simulink model "sampleModel7214_pp_1_1_mu"  (R2018a)
settings: Solver=VariableStepAuto  StartTime=0.0  StopTime=10.0  RelTol=1e-3
undefined symbols (not defined in the file): DiscIntNeverNeededParam
libraries: simulink x52
(part 1 of 2)
settings Model: Creator=cyfuzz  LastModifiedBy=shafiul
settings CodeAppCC: StateflowObjectComments=on

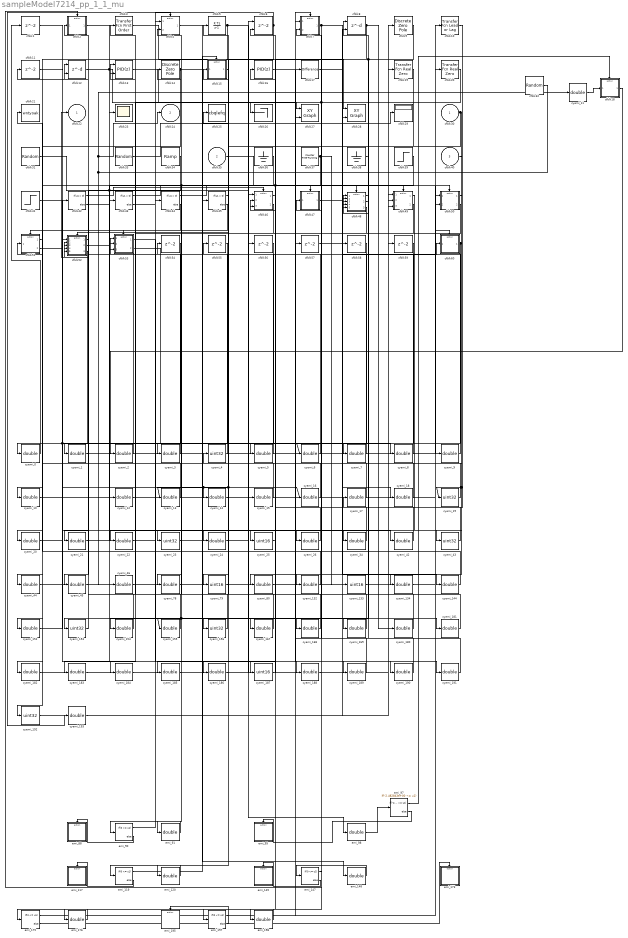
== system sampleModel7214_pp_1_1_mu ==
  cfblk30 : Inport
  cfblk35 : Inport  Port=2
  cfblk40 : Inport  Port=3
  cfblk{1,11,54..59} (8 alike) : Delay  SampleTime=1
  cfblk10 : simulink/Discrete/Transfer Fcn Lead or Lag  PoleZ=0.95  ZeroZ=0.75  ICPrevOutput=0.0  ICPrevInput=0.0  DoSatur=off
      settings: SourceProductName=Simulink  SourceProductBaseCode=SL
  cfblk12 : Delay  DelayLengthSource=Input port  SampleTime=1
      settings: InputPortMap=u0,p1
  cfblk13 : simulink/Continuous/PID Controller (2DOF)  Controller=PID  TimeDomain=Discrete-time  SampleTime=1  IntegratorMethod=Forward Euler  FilterMethod=Forward Euler  Form=Parallel  UseFilter=on  ControllerParametersSource=internal  P=1  I=1  D=0  N=100  b=1  c=1  InitialConditionSource=internal  InitialConditionForIntegrator=0  InitialConditionForFilter=0  ExternalReset=none  LimitOutput=off  UpperSaturationLimit=inf  LowerSaturationLimit=-inf  LinearizeAsGain=off  AntiWindupMode=none  Kb=1  TrackingMode=off  Kt=1  PParamMin=[]  PParamMax=[]  IParamMin=[]  IParamMax=[]  DParamMin=[]  DParamMax=[]  NParamMin=[]  NParamMax=[]  bParamMin=[]  bParamMax=[]  cParamMin=[]  cParamMax=[]  KbParamMin=[]  KbParamMax=[]  KtParamMin=[]  KtParamMax=[]  POutMin=[]  POutMax=[]  IOutMin=[]  IOutMax=[]  DOutMin=[]  DOutMax=[]  NOutMin=[]  NOutMax=[]  bOutMin=[]  bOutMax=[]  cOutMin=[]  cOutMax=[]  KbOutMin=[]  KbOutMax=[]  KtOutMin=[]  KtOutMax=[]  IntegratorOutMin=[]  IntegratorOutMax=[]  FilterOutMin=[]  FilterOutMax=[]  SumOutMin=[]  SumOutMax=[]  Sum1OutMin=[]  Sum1OutMax=[]  Sum2OutMin=[]  Sum2OutMax=[]  Sum3OutMin=[]  Sum3OutMax=[]  SumI1OutMin=[]  SumI1OutMax=[]  SumI2OutMin=[]  SumI2OutMax=[]  SumI3OutMin=[]  SumI3OutMax=[]  SumDOutMin=[]  SumDOutMax=[]  SaturationOutMin=[]  SaturationOutMax=[]  IntegratorContinuousStateAttributes=''  IntegratorStateMustResolveToSignalObject=off  IntegratorRTWStateStorageClass=Auto  FilterContinuousStateAttributes=''  FilterStateMustResolveToSignalObject=off  FilterRTWStateStorageClass=Auto  DifferentiatorICPrevScaledInput=0  DifferentiatorOutMin=[]  DifferentiatorOutMax=[]  FilterDiffOutCoefMin=[]  FilterDiffOutCoefMax=[]  SumDenOutMin=[]  SumDenOutMax=[]  SumNumOutMin=[]  SumNumOutMax=[]  ReciprocalOutMin=[]  ReciprocalOutMax=[]  DivideOutMin=[]  DivideOutMax=[]  TunerSelectOption=Transfer Function Based (PID Tuner App)
  cfblk14 : DiscreteZeroPole  Poles=[0 0.5]  Gain=1
  cfblk15 : Subsystem  TreatAsAtomicUnit=on
  cfblk16 : simulink/Continuous/PID Controller  Controller=PID  TimeDomain=Discrete-time  SampleTime=1  IntegratorMethod=Forward Euler  FilterMethod=Forward Euler  Form=Parallel  UseFilter=on  ControllerParametersSource=internal  P=1  I=1  D=0  N=100  InitialConditionSource=internal  InitialConditionForIntegrator=0  InitialConditionForFilter=0  ExternalReset=none  LimitOutput=off  UpperSaturationLimit=inf  LowerSaturationLimit=-inf  LinearizeAsGain=off  AntiWindupMode=none  Kb=1  TrackingMode=off  Kt=1  PParamMin=[]  PParamMax=[]  IParamMin=[]  IParamMax=[]  DParamMin=[]  DParamMax=[]  NParamMin=[]  NParamMax=[]  KbParamMin=[]  KbParamMax=[]  KtParamMin=[]  KtParamMax=[]  POutMin=[]  POutMax=[]  IOutMin=[]  IOutMax=[]  DOutMin=[]  DOutMax=[]  NOutMin=[]  NOutMax=[]  KbOutMin=[]  KbOutMax=[]  KtOutMin=[]  KtOutMax=[]  IntegratorOutMin=[]  IntegratorOutMax=[]  FilterOutMin=[]  FilterOutMax=[]  SumOutMin=[]  SumOutMax=[]  SumI1OutMin=[]  SumI1OutMax=[]  SumI2OutMin=[]  SumI2OutMax=[]  SumI3OutMin=[]  SumI3OutMax=[]  SumDOutMin=[]  SumDOutMax=[]  SaturationOutMin=[]  SaturationOutMax=[]  IntegratorContinuousStateAttributes=''  IntegratorStateMustResolveToSignalObject=off  IntegratorRTWStateStorageClass=Auto  FilterContinuousStateAttributes=''  FilterStateMustResolveToSignalObject=off  FilterRTWStateStorageClass=Auto  DifferentiatorICPrevScaledInput=0  DifferentiatorOutMin=[]  DifferentiatorOutMax=[]  FilterDiffOutCoefMin=[]  FilterDiffOutCoefMax=[]  SumDenOutMin=[]  SumDenOutMax=[]  SumNumOutMin=[]  SumNumOutMax=[]  ReciprocalOutMin=[]  ReciprocalOutMax=[]  DivideOutMin=[]  DivideOutMax=[]  TunerSelectOption=Transfer Function Based (PID Tuner App)
  cfblk17 : simulink/Discrete/Difference  ICPrevInput=0.0  OutMin=[]  OutMax=[]  OutDataTypeStr=double  OutputDataTypeScalingMode=double  OutDataType=fixdt(1, 16)  OutScaling=2^-10  DoSatur=off
  cfblk18 : Subsystem  TreatAsAtomicUnit=on
  cfblk19 : simulink/Discrete/Transfer Fcn Real Zero  ZeroZ=0.75  ICPrevInput=0.0  DoSatur=off
      settings: SourceProductName=Simulink  SourceProductBaseCode=SL
  cfblk2 : Subsystem  TreatAsAtomicUnit=on
  cfblk20 : simulink/Discrete/Transfer Fcn Real Zero  ZeroZ=0.75  ICPrevInput=0.0  DoSatur=off
      settings: SourceProductName=Simulink  SourceProductBaseCode=SL
  cfblk21 : ToWorkspace  VariableName=wntyoak  SaveFormat=Timeseries  SampleTime=-1
  cfblk23 : Scope
  cfblk25 : ToWorkspace  VariableName=cbqlefq  SaveFormat=Timeseries  SampleTime=-1
  cfblk26 : Terminator
  cfblk27 : simulink/Sinks/XY Graph  xmin=-1  xmax=1  ymin=-1  ymax=1  st=-1
  cfblk28 : simulink/Sinks/XY Graph  xmin=-1  xmax=1  ymin=-1  ymax=1  st=-1
  cfblk29 : Display
  cfblk3 : simulink/Discrete/Transfer Fcn First Order  PoleZ=0.95  ICPrevOutput=0.0  DoSatur=off
      settings: SourceProductName=Simulink
  cfblk31 : RandomNumber  SampleTime=0.1
  cfblk32 : RandomNumber  SampleTime=0.1
  cfblk33 : UniformRandomNumber  SampleTime=0.1
  cfblk34 : simulink/Sources/Ramp  slope=1  start=0  InitialOutput=0
  cfblk36 : Ground
  cfblk37 : simulink/Sources/Counter Free-Running  NumBits=16  tsamp=1
  cfblk38 : Ground
  cfblk39 : Step  After=69  SampleTime=0
  cfblk4 : Subsystem  TreatAsAtomicUnit=on
  cfblk41 : Step  After=79  SampleTime=0
  cfblk{42..45} (4 alike) : If  SampleTime=1
  cfblk46 : Subsystem  TreatAsAtomicUnit=on
  cfblk47 : Subsystem  TreatAsAtomicUnit=on
  cfblk48 : Subsystem  TreatAsAtomicUnit=on
  cfblk49 : Subsystem  TreatAsAtomicUnit=on
  cfblk5 : DiscreteIntegrator  OutDataTypeStr=double  ICPrevOutput=DiscIntNeverNeededParam  ICPrevScaledInput=DiscIntNeverNeededParam
  cfblk50 : Subsystem  TreatAsAtomicUnit=on
  cfblk51 : Subsystem  TreatAsAtomicUnit=on
  cfblk52 : Subsystem  TreatAsAtomicUnit=on
  cfblk53 : Subsystem  TreatAsAtomicUnit=on
  cfblk6 : Delay  ShowEnablePort=on  SampleTime=1
      settings: InputPortMap=u0,e6
  cfblk60 : Subsystem  TreatAsAtomicUnit=on
  cfblk7 : Subsystem  TreatAsAtomicUnit=on
  cfblk8 : Delay  DelayLengthSource=Input port  SampleTime=1
      settings: InputPortMap=u0,p1
  cfblk9 : DiscreteZeroPole  Poles=[0 0.5]  Gain=1
  cyemi_{0..3,5..18,20..22,24,26,34,42,44..46,78,80,132,134,144,152,154..155,167..169,180..186,188..191,193} (51 alike) : DataTypeConversion  OutDataTypeStr=double
  cyemi_{25,79,133,187} (4 alike) : DataTypeConversion  OutDataTypeStr=uint16
  cyemi_{4,19,23,43,153,156,192} (7 alike) : DataTypeConversion  OutDataTypeStr=uint32
  emi_117 : Subsystem  TreatAsAtomicUnit=on
  emi_{90,119,147,175,197} (5 alike) : If  IfExpression=0 <= u1
  emi_{91,98,120,148,176,198} (6 alike) : DataTypeConversion  OutDataTypeStr=double
  emi_145 : Subsystem  TreatAsAtomicUnit=on
  emi_173 : Subsystem  TreatAsAtomicUnit=on
  emi_195 : Subsystem  TreatAsAtomicUnit=on
  emi_88 : Subsystem  TreatAsAtomicUnit=on
  emi_95 : Subsystem  TreatAsAtomicUnit=on
  emi_97 : If  IfExpression=-2.482843e+00 <= u1  SampleTime=1
  cfblk22 : Outport
  cfblk24 : Outport  Port=2
  wires:
  cfblk52/1(cfblk2) -> cfblk22/1
  cfblk37/1 -> cyemi_79/1, cyemi_187/1, cyemi_133/1
  cfblk3/1 -> cfblk28/1
  cfblk13/1 -> cfblk26/1
  cfblk20/1 -> cyemi_132/1, cyemi_154/1
  cfblk32/1 -> cyemi_11/1, cfblk24/1, cyemi_46/1
  cfblk9/1 -> cyemi_5/1, cyemi_7/1
  cfblk8/1 -> cfblk27/1, cyemi_180/1
  cfblk36/1 -> cyemi_23/1, cyemi_192/1
  cfblk41/1 -> cyemi_14/1, cyemi_16/1, cyemi_6/1
  cfblk5/1 -> cyemi_34/1, cyemi_44/1
  cfblk12/1 -> cfblk27/2, cyemi_188/1
  cfblk33/1 -> cfblk29/1
  cfblk30/1 -> cyemi_19/1, cyemi_43/1, cyemi_156/1
  cfblk42/1 -> cfblk46/Action
  cfblk42/2 -> cfblk47/Action
  cfblk43/1 -> cfblk48/Action
  cfblk43/2 -> cfblk49/Action
  cfblk44/1 -> cfblk50/Action
  cfblk44/2 -> cfblk51/Action
  cfblk45/1 -> cfblk52/Action
  cfblk45/2 -> cfblk53/Action
  cyemi_0/1 -> cfblk1/1
  cfblk58/1 -> cyemi_0/1
  cyemi_1/1 -> cfblk10/1
  cfblk34/1 -> cyemi_1/1
  cyemi_2/1 -> cfblk11/1
  cyemi_3/1 -> cfblk12/1
  cfblk51/2(cfblk8) -> cyemi_3/1
  cyemi_4/1 -> cfblk12/2
  cfblk40/1 -> cyemi_4/1
  cyemi_5/1 -> cfblk13/1
  cyemi_6/1 -> cfblk13/2
  cyemi_7/1 -> cfblk14/1
  cyemi_9/1 -> cfblk16/1
  cfblk35/1 -> cyemi_9/1
  cyemi_10/1 -> cfblk17/1
  cfblk51/1(cfblk2) -> cyemi_10/1
  cyemi_12/1 -> cfblk19/1
  cfblk31/1 -> cyemi_12/1, emi_98/1
  cyemi_14/1 -> cfblk20/1
  cyemi_15/1 -> cfblk21/1
  cfblk53/2(cfblk11) -> cyemi_15/1
  cyemi_16/1 -> cfblk25/1
  cyemi_17/1 -> cfblk3/1
  cfblk10/1 -> cyemi_17/1
  cfblk17/1 -> cyemi_18/1
  cyemi_20/1 -> cfblk42/1
  cfblk52/3(cfblk15) -> cyemi_20/1
  cyemi_21/1 -> cfblk43/1
  cfblk55/1 -> cyemi_21/1
  cyemi_22/1 -> cfblk44/1
  cfblk49/1(cfblk2) -> cyemi_22/1
  cyemi_23/1 -> cfblk45/1
  cyemi_24/1 -> cfblk46/1(cfblk1)
  cfblk49/2(cfblk16) -> cyemi_24/1
  cyemi_25/1 -> cfblk46/2(cfblk9)
  cfblk50/1(cfblk2) -> cyemi_25/1
  cyemi_26/1 -> cfblk46/3(cfblk10)
  cfblk19/1 -> cyemi_26/1
  cyemi_34/1 -> cfblk47/1(cfblk1)
  cyemi_42/1 -> cfblk48/1(cfblk1)
  cfblk1/1 -> cyemi_42/1
  cyemi_43/1 -> cfblk48/2(cfblk10)
  cyemi_44/1 -> cfblk48/3(cfblk11)
  cyemi_45/1 -> cfblk48/4(cfblk12)
  cfblk54/1 -> cyemi_45/1
  cyemi_46/1 -> cfblk48/5(cfblk13)
  cyemi_78/1 -> cfblk49/1(cfblk1)
  cfblk48/3(cfblk15) -> cyemi_78/1
  cyemi_79/1 -> cfblk49/2(cfblk14)
  cyemi_80/1 -> cfblk49/3(cfblk15)
  cyemi_132/1 -> cfblk5/1
  cyemi_133/1 -> cfblk50/1(cfblk1)
  cyemi_134/1 -> cfblk50/2(cfblk12)
  cfblk57/1 -> cyemi_134/1
  cyemi_144/1 -> cfblk51/1(cfblk1)
  cfblk47/1(cfblk2) -> cyemi_144/1
  cyemi_152/1 -> cfblk52/1(cfblk1)
  cfblk56/1 -> cyemi_152/1
  cyemi_153/1 -> cfblk52/2(cfblk10)
  cfblk48/2(cfblk14) -> cyemi_153/1
  cyemi_154/1 -> cfblk52/3(cfblk11)
  cyemi_155/1 -> cfblk52/4(cfblk12)
  cfblk59/1 -> cyemi_155/1, emi_91/1
  cyemi_156/1 -> cfblk52/5(cfblk13)
  cyemi_167/1 -> cfblk53/1(cfblk1)
  cfblk48/1(cfblk2) -> cyemi_167/1
  cyemi_168/1 -> cfblk53/2(cfblk9)
  cfblk39/1 -> cyemi_168/1
  cyemi_169/1 -> cfblk53/3(cfblk10)
  cfblk38/1 -> cyemi_169/1
  cyemi_180/1 -> cfblk54/1
  cyemi_181/1 -> cfblk55/1
  cfblk52/2(cfblk14) -> cyemi_181/1
  cyemi_182/1 -> cfblk56/1
  cfblk14/1 -> cyemi_182/1, emi_148/1
  cyemi_183/1 -> cfblk57/1
  cfblk46/2(cfblk11) -> cyemi_183/1
  cyemi_184/1 -> cfblk58/1
  cfblk50/2(cfblk13) -> cyemi_184/1
  cyemi_185/1 -> cfblk59/1
  cyemi_186/1 -> cfblk6/1
  cfblk46/1(cfblk2) -> cyemi_186/1
  cyemi_187/1 -> cfblk6/2
  cfblk11/1 -> cyemi_189/1
  cfblk16/1 -> cyemi_190/1
  cyemi_191/1 -> cfblk8/1
  cfblk53/1(cfblk2) -> cyemi_191/1
  cyemi_192/1 -> cfblk8/2
  cyemi_193/1 -> cfblk9/1
  cfblk6/1 -> cyemi_193/1, emi_120/1
  cyemi_18/1 -> cfblk4/1(emi_85)
  cyemi_19/1 -> cfblk4/2(emi_86)
  cfblk4/1(emi_87) -> cyemi_8/1
  emi_90/1 -> cfblk4/Action
  emi_90/2 -> emi_88/Action
  emi_91/1 -> emi_90/1
  cyemi_11/1 -> cfblk18/1(emi_93)
  cfblk18/1(emi_94) -> cyemi_2/1
  emi_97/1 -> cfblk18/Action
  emi_97/2 -> emi_95/Action
  emi_98/1 -> emi_97/1
  cyemi_8/1 -> cfblk15/1(emi_115)
  cfblk15/1(emi_116) -> cyemi_185/1, cyemi_13/1
  emi_119/1 -> cfblk15/Action
  emi_119/2 -> emi_117/Action
  emi_120/1 -> emi_119/1
  cyemi_13/1 -> cfblk2/1(emi_143)
  cfblk2/1(emi_144) -> cfblk23/1
  emi_147/1 -> cfblk2/Action
  emi_147/2 -> emi_145/Action
  emi_148/1 -> emi_147/1
  cyemi_188/1 -> cfblk60/1(emi_171)
  cfblk60/1(emi_172) -> cyemi_80/1, emi_198/1
  emi_175/1 -> cfblk60/Action
  emi_175/2 -> emi_173/Action
  emi_176/1 -> emi_175/1
  cyemi_189/1 -> cfblk7/1(emi_192)
  cyemi_190/1 -> cfblk7/2(emi_193)
  cfblk7/1(emi_194) -> emi_176/1, cfblk28/2
  emi_197/1 -> cfblk7/Action
  emi_197/2 -> emi_195/Action
  emi_198/1 -> emi_197/1

== system sampleModel7214_pp_1_1_mu/cfblk15 ==
  emi_115 : Inport
  Action Port : ActionPort  ActionType=then
  cfblk15 : simulink/Discrete/Transfer Fcn Real Zero  ZeroZ=0.75  ICPrevInput=0.0  DoSatur=off
      settings: SourceProductName=Simulink  SourceProductBaseCode=SL
  emi_116 : Outport
  wires:
  emi_115/1 -> cfblk15/1
  cfblk15/1 -> emi_116/1

== system sampleModel7214_pp_1_1_mu/cfblk18 ==
  emi_93 : Inport
  Action Port : ActionPort  ActionType=then
  cfblk18 : UnitDelay
  emi_94 : Outport
  wires:
  emi_93/1 -> cfblk18/1
  cfblk18/1 -> emi_94/1

== system sampleModel7214_pp_1_1_mu/cfblk2 ==
  emi_143 : Inport
  Action Port : ActionPort  ActionType=then
  cfblk2 : simulink/Discrete/Difference  ICPrevInput=0.0  OutMin=[]  OutMax=[]  OutDataTypeStr=double  OutputDataTypeScalingMode=double  OutDataType=fixdt(1, 16)  OutScaling=2^-10  DoSatur=off
  emi_144 : Outport
  wires:
  emi_143/1 -> cfblk2/1
  cfblk2/1 -> emi_144/1

== system sampleModel7214_pp_1_1_mu/cfblk4 ==
  emi_85 : Inport
  emi_86 : Inport  Port=2
  Action Port : ActionPort  ActionType=then
  cfblk4 : Delay  ShowEnablePort=on  SampleTime=1
      settings: InputPortMap=u0,e6
  emi_87 : Outport
  wires:
  emi_85/1 -> cfblk4/1
  emi_86/1 -> cfblk4/2
  cfblk4/1 -> emi_87/1

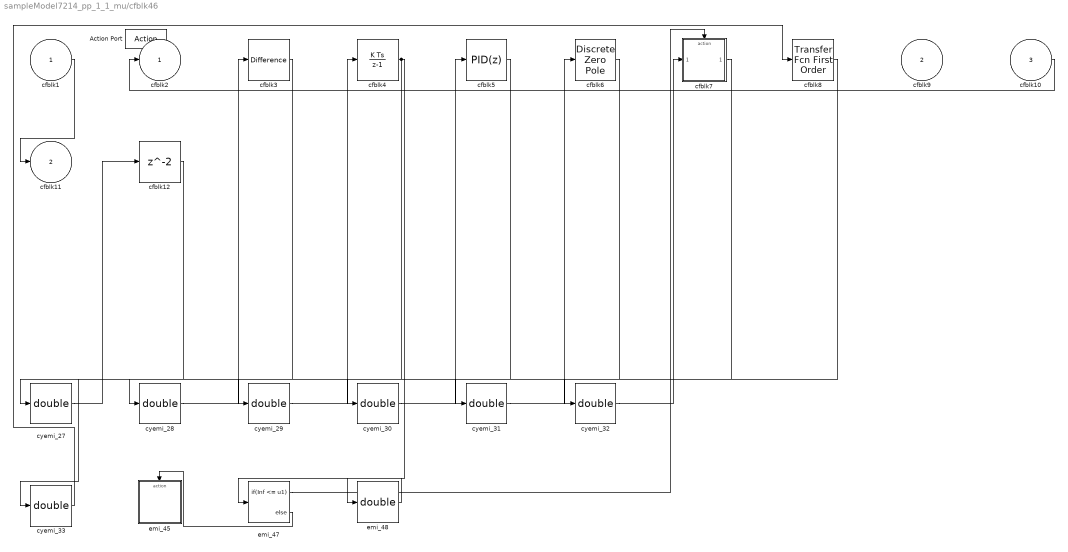
== system sampleModel7214_pp_1_1_mu/cfblk46 ==
  cfblk1 : Inport
  cfblk9 : Inport  Port=2
  cfblk10 : Inport  Port=3
  Action Port : ActionPort  ActionType=then
  cfblk12 : Delay
  cfblk3 : simulink/Discrete/Difference  ICPrevInput=0.0  OutMin=[]  OutMax=[]  OutDataTypeStr=double  OutputDataTypeScalingMode=double  OutDataType=fixdt(1, 16)  OutScaling=2^-10  DoSatur=off
  cfblk4 : DiscreteIntegrator  SampleTime=-1  OutDataTypeStr=double  ICPrevOutput=DiscIntNeverNeededParam  ICPrevScaledInput=DiscIntNeverNeededParam
  cfblk5 : simulink/Continuous/PID Controller  Controller=PID  TimeDomain=Discrete-time  SampleTime=-1  IntegratorMethod=Forward Euler  FilterMethod=Forward Euler  Form=Parallel  UseFilter=on  ControllerParametersSource=internal  P=1  I=1  D=0  N=100  InitialConditionSource=internal  InitialConditionForIntegrator=0  InitialConditionForFilter=0  ExternalReset=none  LimitOutput=off  UpperSaturationLimit=inf  LowerSaturationLimit=-inf  LinearizeAsGain=off  AntiWindupMode=none  Kb=1  TrackingMode=off  Kt=1  PParamMin=[]  PParamMax=[]  IParamMin=[]  IParamMax=[]  DParamMin=[]  DParamMax=[]  NParamMin=[]  NParamMax=[]  KbParamMin=[]  KbParamMax=[]  KtParamMin=[]  KtParamMax=[]  POutMin=[]  POutMax=[]  IOutMin=[]  IOutMax=[]  DOutMin=[]  DOutMax=[]  NOutMin=[]  NOutMax=[]  KbOutMin=[]  KbOutMax=[]  KtOutMin=[]  KtOutMax=[]  IntegratorOutMin=[]  IntegratorOutMax=[]  FilterOutMin=[]  FilterOutMax=[]  SumOutMin=[]  SumOutMax=[]  SumI1OutMin=[]  SumI1OutMax=[]  SumI2OutMin=[]  SumI2OutMax=[]  SumI3OutMin=[]  SumI3OutMax=[]  SumDOutMin=[]  SumDOutMax=[]  SaturationOutMin=[]  SaturationOutMax=[]  IntegratorContinuousStateAttributes=''  IntegratorStateMustResolveToSignalObject=off  IntegratorRTWStateStorageClass=Auto  FilterContinuousStateAttributes=''  FilterStateMustResolveToSignalObject=off  FilterRTWStateStorageClass=Auto  DifferentiatorICPrevScaledInput=0  DifferentiatorOutMin=[]  DifferentiatorOutMax=[]  FilterDiffOutCoefMin=[]  FilterDiffOutCoefMax=[]  SumDenOutMin=[]  SumDenOutMax=[]  SumNumOutMin=[]  SumNumOutMax=[]  ReciprocalOutMin=[]  ReciprocalOutMax=[]  DivideOutMin=[]  DivideOutMax=[]  TunerSelectOption=Transfer Function Based (PID Tuner App)
  cfblk6 : DiscreteZeroPole  Poles=[0 0.5]  Gain=1  SampleTime=-1
  cfblk7 : Subsystem  TreatAsAtomicUnit=on
  cfblk8 : simulink/Discrete/Transfer Fcn First Order  PoleZ=0.95  ICPrevOutput=0.0  DoSatur=off
      settings: SourceProductName=Simulink
  cyemi_{27..33} (7 alike) : DataTypeConversion  OutDataTypeStr=double
  emi_45 : Subsystem  TreatAsAtomicUnit=on
  emi_47 : If  IfExpression=Inf <= u1
  emi_48 : DataTypeConversion  OutDataTypeStr=double
  cfblk2 : Outport
  cfblk11 : Outport  Port=2
  wires:
  cfblk10/1 -> cfblk2/1
  cfblk1/1 -> cfblk11/1
  cyemi_27/1 -> cfblk12/1
  cfblk5/1 -> cyemi_27/1
  cyemi_28/1 -> cfblk3/1
  cfblk12/1 -> cyemi_28/1
  cyemi_29/1 -> cfblk4/1
  cyemi_30/1 -> cfblk5/1
  cfblk4/1 -> cyemi_30/1, emi_48/1
  cyemi_31/1 -> cfblk6/1
  cfblk8/1 -> cyemi_31/1
  cfblk6/1 -> cyemi_32/1
  cyemi_33/1 -> cfblk8/1
  cfblk3/1 -> cyemi_33/1
  cyemi_32/1 -> cfblk7/1(emi_43)
  cfblk7/1(emi_44) -> cyemi_29/1
  emi_47/1 -> cfblk7/Action
  emi_47/2 -> emi_45/Action
  emi_48/1 -> emi_47/1

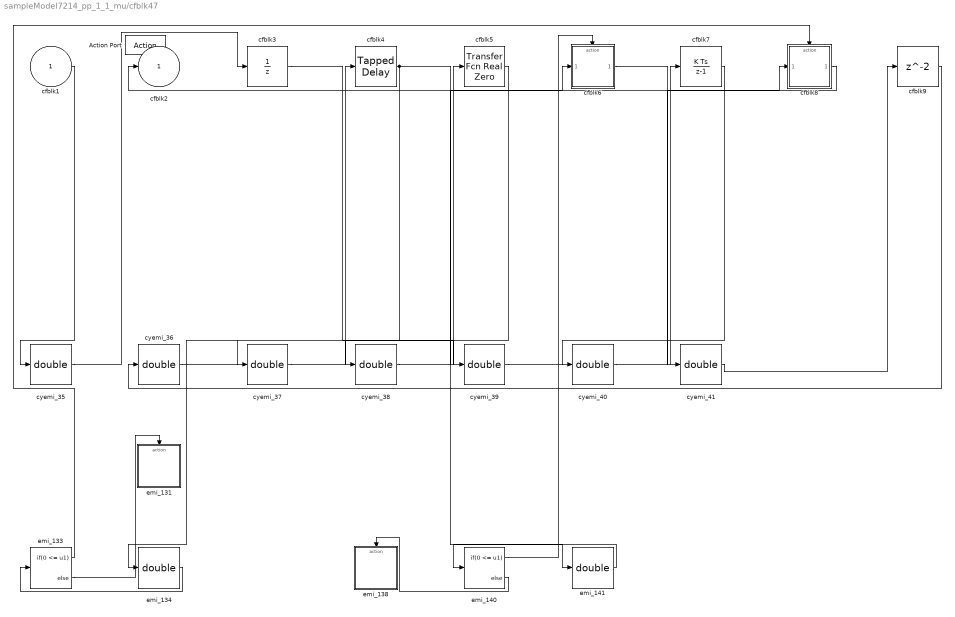
== system sampleModel7214_pp_1_1_mu/cfblk47 ==
  cfblk1 : Inport
  Action Port : ActionPort  ActionType=else
  cfblk3 : UnitDelay  SampleTime=-1
  cfblk4 : simulink/Discrete/Tapped Delay  vinit=0.0  samptime=-1  NumDelays=1  DelayOrder=Oldest  includeCurrent=off
  cfblk5 : simulink/Discrete/Transfer Fcn Real Zero  ZeroZ=0.75  ICPrevInput=0.0  DoSatur=off
      settings: SourceProductName=Simulink  SourceProductBaseCode=SL
  cfblk6 : Subsystem  TreatAsAtomicUnit=on
  cfblk7 : DiscreteIntegrator  SampleTime=-1  OutDataTypeStr=double  ICPrevOutput=DiscIntNeverNeededParam  ICPrevScaledInput=DiscIntNeverNeededParam
  cfblk8 : Subsystem  TreatAsAtomicUnit=on
  cfblk9 : Delay
  cyemi_{35..41} (7 alike) : DataTypeConversion  OutDataTypeStr=double
  emi_131 : Subsystem  TreatAsAtomicUnit=on
  emi_133 : If  IfExpression=0 <= u1
  emi_134 : DataTypeConversion  OutDataTypeStr=double
  emi_138 : Subsystem  TreatAsAtomicUnit=on
  emi_140 : If  IfExpression=0 <= u1
  emi_141 : DataTypeConversion  OutDataTypeStr=double
  cfblk2 : Outport
  wires:
  cyemi_35/1 -> cfblk3/1
  cfblk1/1 -> cyemi_35/1
  cyemi_36/1 -> cfblk4/1
  cfblk9/1 -> cyemi_36/1
  cyemi_37/1 -> cfblk5/1
  cfblk4/1 -> cyemi_37/1, emi_134/1, emi_141/1
  cfblk5/1 -> cyemi_38/1
  cyemi_39/1 -> cfblk7/1
  cfblk3/1 -> cyemi_39/1
  cfblk7/1 -> cyemi_40/1
  cyemi_41/1 -> cfblk9/1
  cyemi_40/1 -> cfblk8/1(emi_129)
  cfblk8/1(emi_130) -> cfblk2/1
  emi_133/1 -> cfblk8/Action
  emi_133/2 -> emi_131/Action
  emi_134/1 -> emi_133/1
  cyemi_38/1 -> cfblk6/1(emi_136)
  cfblk6/1(emi_137) -> cyemi_41/1
  emi_140/1 -> cfblk6/Action
  emi_140/2 -> emi_138/Action
  emi_141/1 -> emi_140/1

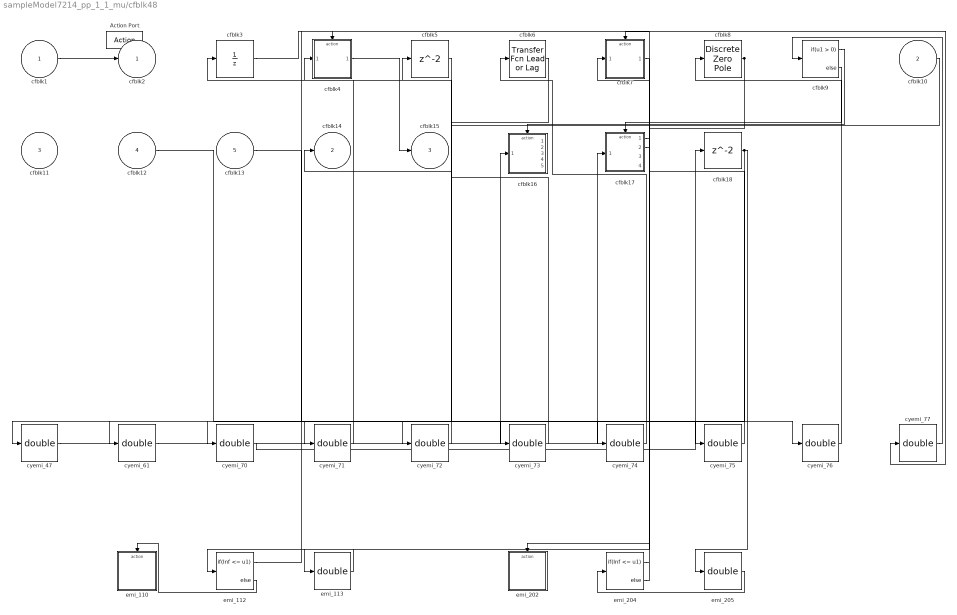
== system sampleModel7214_pp_1_1_mu/cfblk48 ==
  cfblk1 : Inport
  cfblk10 : Inport  Port=2
  cfblk11 : Inport  Port=3
  cfblk12 : Inport  Port=4
  cfblk13 : Inport  Port=5
  Action Port : ActionPort  ActionType=then
  cfblk16 : Subsystem  TreatAsAtomicUnit=on
  cfblk17 : Subsystem  TreatAsAtomicUnit=on
  cfblk18 : Delay
  cfblk3 : UnitDelay  SampleTime=-1
  cfblk4 : Subsystem  TreatAsAtomicUnit=on
  cfblk5 : Delay
  cfblk6 : simulink/Discrete/Transfer Fcn Lead or Lag  PoleZ=0.95  ZeroZ=0.75  ICPrevOutput=0.0  ICPrevInput=0.0  DoSatur=off
      settings: SourceProductName=Simulink  SourceProductBaseCode=SL
  cfblk7 : Subsystem  TreatAsAtomicUnit=on
  cfblk8 : DiscreteZeroPole  Poles=[0 0.5]  Gain=1  SampleTime=-1
  cfblk9 : If  SampleTime=1
  cyemi_{47,61,70..77} (10 alike) : DataTypeConversion  OutDataTypeStr=double
  emi_110 : Subsystem  TreatAsAtomicUnit=on
  emi_112 : If  IfExpression=Inf <= u1
  emi_113 : DataTypeConversion  OutDataTypeStr=double
  emi_202 : Subsystem  TreatAsAtomicUnit=on
  emi_204 : If  IfExpression=Inf <= u1
  emi_205 : DataTypeConversion  OutDataTypeStr=double
  cfblk2 : Outport
  cfblk14 : Outport  Port=2
  cfblk15 : Outport  Port=3
  wires:
  cfblk10/1 -> cfblk14/1
  cfblk1/1 -> cfblk2/1
  cfblk9/1 -> cfblk16/Action
  cfblk9/2 -> cfblk17/Action
  cyemi_47/1 -> cfblk16/1(cfblk1)
  cfblk17/1(cfblk2) -> cyemi_47/1
  cyemi_61/1 -> cfblk17/1(cfblk1)
  cfblk8/1 -> cyemi_61/1, emi_113/1
  cyemi_70/1 -> cfblk18/1
  cfblk5/1 -> cyemi_70/1
  cyemi_71/1 -> cfblk3/1
  cfblk18/1 -> cyemi_71/1, emi_205/1
  cfblk6/1 -> cyemi_72/1
  cyemi_73/1 -> cfblk5/1
  cfblk17/2(cfblk9) -> cyemi_73/1
  cyemi_74/1 -> cfblk6/1
  cfblk12/1 -> cyemi_75/1
  cyemi_76/1 -> cfblk8/1
  cfblk13/1 -> cyemi_76/1
  cyemi_77/1 -> cfblk9/1
  cfblk3/1 -> cyemi_77/1
  cyemi_72/1 -> cfblk4/1(emi_108)
  cfblk4/1(emi_109) -> cfblk15/1
  emi_112/1 -> cfblk4/Action
  emi_112/2 -> emi_110/Action
  emi_113/1 -> emi_112/1
  cyemi_75/1 -> cfblk7/1(emi_200)
  cfblk7/1(emi_201) -> cyemi_74/1
  emi_204/1 -> cfblk7/Action
  emi_204/2 -> emi_202/Action
  emi_205/1 -> emi_204/1

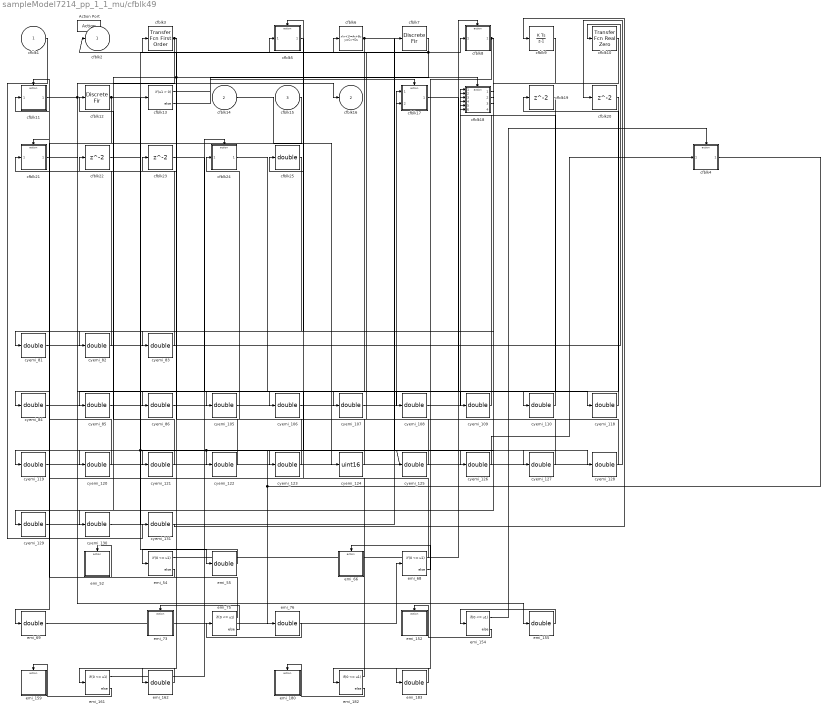
== system sampleModel7214_pp_1_1_mu/cfblk49 ==
  cfblk1 : Inport
  cfblk14 : Inport  Port=2
  cfblk15 : Inport  Port=3
  Action Port : ActionPort  ActionType=else
  cfblk10 : simulink/Discrete/Transfer Fcn Real Zero  ZeroZ=0.75  ICPrevInput=0.0  DoSatur=off
      settings: SourceProductName=Simulink  SourceProductBaseCode=SL
  cfblk11 : Subsystem  TreatAsAtomicUnit=on
  cfblk12 : DiscreteFir
  cfblk13 : If  SampleTime=1
  cfblk17 : Subsystem  TreatAsAtomicUnit=on
  cfblk18 : Subsystem  TreatAsAtomicUnit=on
  cfblk{19..20,22..23} (4 alike) : Delay
  cfblk21 : Subsystem  TreatAsAtomicUnit=on
  cfblk24 : Subsystem  TreatAsAtomicUnit=on
  cfblk25 : DataTypeConversion  OutDataTypeStr=double
  cfblk3 : simulink/Discrete/Transfer Fcn First Order  PoleZ=0.95  ICPrevOutput=0.0  DoSatur=off
      settings: SourceProductName=Simulink
  cfblk4 : Subsystem  TreatAsAtomicUnit=on
  cfblk5 : Subsystem  TreatAsAtomicUnit=on
  cfblk6 : DiscreteStateSpace  SampleTime=-1
  cfblk7 : DiscreteFir
  cfblk8 : Subsystem  TreatAsAtomicUnit=on
  cfblk9 : DiscreteIntegrator  SampleTime=-1  OutDataTypeStr=double  ICPrevOutput=DiscIntNeverNeededParam  ICPrevScaledInput=DiscIntNeverNeededParam
  cyemi_{81..86,105..110,118..123,125..131} (25 alike) : DataTypeConversion  OutDataTypeStr=double
  cyemi_124 : DataTypeConversion  OutDataTypeStr=uint16
  emi_152 : Subsystem  TreatAsAtomicUnit=on
  emi_{54,68,75,154,161,182} (6 alike) : If  IfExpression=0 <= u1
  emi_{55,69,76,155,162,183} (6 alike) : DataTypeConversion  OutDataTypeStr=double
  emi_159 : Subsystem  TreatAsAtomicUnit=on
  emi_180 : Subsystem  TreatAsAtomicUnit=on
  emi_52 : Subsystem  TreatAsAtomicUnit=on
  emi_66 : Subsystem  TreatAsAtomicUnit=on
  emi_73 : Subsystem  TreatAsAtomicUnit=on
  cfblk2 : Outport
  cfblk16 : Outport  Port=2
  wires:
  cfblk6/1 -> cyemi_123/1, cyemi_127/1
  cfblk3/1 -> cyemi_121/1, cyemi_130/1
  cfblk12/1 -> cyemi_122/1, cyemi_125/1, emi_55/1, emi_69/1
  cfblk7/1 -> cyemi_120/1, emi_162/1, cfblk2/1
  cfblk13/1 -> cfblk17/Action
  cfblk13/2 -> cfblk18/Action
  cyemi_81/1 -> cfblk10/1
  cfblk18/2(cfblk13) -> cyemi_81/1
  cfblk25/1 -> cyemi_82/1
  cyemi_83/1 -> cfblk12/1
  cyemi_84/1 -> cfblk13/1
  cfblk15/1 -> cyemi_84/1
  cyemi_85/1 -> cfblk17/1(cfblk1)
  cfblk18/1(cfblk2) -> cyemi_85/1
  cyemi_86/1 -> cfblk17/2(cfblk15)
  cfblk20/1 -> cyemi_86/1
  cyemi_105/1 -> cfblk18/1(cfblk1)
  cfblk19/1 -> cyemi_105/1
  cyemi_106/1 -> cfblk18/2(cfblk8)
  cfblk9/1 -> cyemi_106/1
  cyemi_107/1 -> cfblk18/3(cfblk9)
  cyemi_108/1 -> cfblk18/4(cfblk10)
  cfblk23/1 -> cyemi_108/1
  cyemi_109/1 -> cfblk18/5(cfblk11)
  cyemi_110/1 -> cfblk18/6(cfblk12)
  cfblk22/1 -> cyemi_110/1
  cyemi_118/1 -> cfblk19/1
  cfblk17/1(cfblk2) -> cyemi_118/1
  cyemi_119/1 -> cfblk20/1
  cfblk10/1 -> cyemi_119/1
  cyemi_121/1 -> cfblk22/1
  cyemi_122/1 -> cfblk23/1
  cyemi_124/1 -> cfblk25/1
  cfblk14/1 -> cyemi_124/1
  cyemi_125/1 -> cfblk3/1
  cfblk18/3(cfblk14) -> cyemi_126/1
  cyemi_128/1 -> cfblk6/1
  cyemi_129/1 -> cfblk7/1
  cyemi_131/1 -> cfblk9/1
  cfblk1/1 -> cyemi_131/1
  cyemi_130/1 -> cfblk8/1(emi_50)
  cfblk8/1(emi_51) -> cyemi_129/1, emi_183/1
  emi_54/1 -> cfblk8/Action
  emi_54/2 -> emi_52/Action
  emi_55/1 -> emi_54/1
  cyemi_120/1 -> cfblk21/1(emi_64)
  cfblk21/1(emi_65) -> cyemi_109/1
  emi_68/1 -> cfblk21/Action
  emi_68/2 -> emi_66/Action
  emi_69/1 -> emi_68/1
  cyemi_82/1 -> cfblk11/1(emi_71)
  cfblk11/1(emi_72) -> cfblk16/1, emi_155/1
  emi_75/1 -> cfblk11/Action
  emi_75/2 -> emi_73/Action
  emi_76/1 -> emi_75/1
  cyemi_126/1 -> cfblk4/1(emi_150)
  cfblk4/1(emi_151) -> cyemi_128/1, emi_76/1
  emi_154/1 -> cfblk4/Action
  emi_154/2 -> emi_152/Action
  emi_155/1 -> emi_154/1
  cyemi_123/1 -> cfblk24/1(emi_157)
  cfblk24/1(emi_158) -> cyemi_107/1
  emi_161/1 -> cfblk24/Action
  emi_161/2 -> emi_159/Action
  emi_162/1 -> emi_161/1
  cyemi_127/1 -> cfblk5/1(emi_178)
  cfblk5/1(emi_179) -> cyemi_83/1
  emi_182/1 -> cfblk5/Action
  emi_182/2 -> emi_180/Action
  emi_183/1 -> emi_182/1

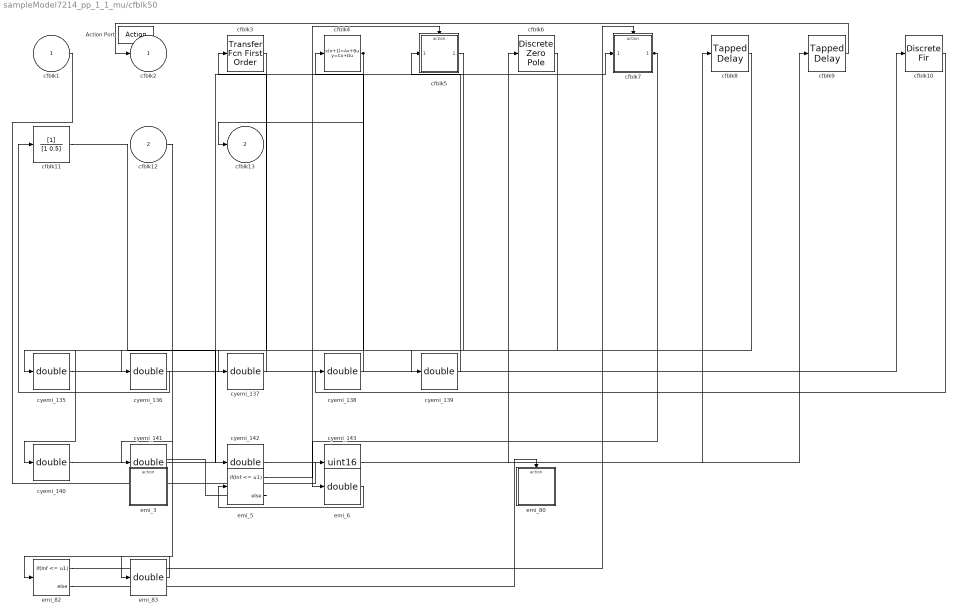
== system sampleModel7214_pp_1_1_mu/cfblk50 ==
  cfblk1 : Inport
  cfblk12 : Inport  Port=2
  Action Port : ActionPort  ActionType=then
  cfblk10 : DiscreteFir
  cfblk11 : DiscreteFilter
  cfblk3 : simulink/Discrete/Transfer Fcn First Order  PoleZ=0.95  ICPrevOutput=0.0  DoSatur=off
      settings: SourceProductName=Simulink
  cfblk4 : DiscreteStateSpace  SampleTime=-1
  cfblk5 : Subsystem  TreatAsAtomicUnit=on
  cfblk6 : DiscreteZeroPole  Poles=[0 0.5]  Gain=1  SampleTime=-1
  cfblk7 : Subsystem  TreatAsAtomicUnit=on
  cfblk8 : simulink/Discrete/Tapped Delay  vinit=0.0  samptime=-1  NumDelays=1  DelayOrder=Oldest  includeCurrent=off
  cfblk9 : simulink/Discrete/Tapped Delay  vinit=0.0  samptime=-1  NumDelays=1  DelayOrder=Oldest  includeCurrent=off
  cyemi_{135..142} (8 alike) : DataTypeConversion  OutDataTypeStr=double
  cyemi_143 : DataTypeConversion  OutDataTypeStr=uint16
  emi_3 : Subsystem  TreatAsAtomicUnit=on
  emi_5 : If  IfExpression=Inf <= u1
  emi_6 : DataTypeConversion  OutDataTypeStr=double
  emi_80 : Subsystem  TreatAsAtomicUnit=on
  emi_82 : If  IfExpression=Inf <= u1
  emi_83 : DataTypeConversion  OutDataTypeStr=double
  cfblk2 : Outport
  cfblk13 : Outport  Port=2
  wires:
  cfblk9/1 -> cfblk2/1
  cfblk4/1 -> cfblk13/1, emi_83/1
  cyemi_135/1 -> cfblk10/1
  cfblk6/1 -> cyemi_135/1
  cyemi_136/1 -> cfblk11/1
  cyemi_137/1 -> cfblk3/1
  cfblk8/1 -> cyemi_137/1
  cyemi_138/1 -> cfblk4/1
  cfblk10/1 -> cyemi_138/1
  cyemi_140/1 -> cfblk6/1
  cfblk3/1 -> cyemi_140/1
  cfblk12/1 -> cyemi_141/1
  cyemi_142/1 -> cfblk8/1
  cfblk11/1 -> cyemi_142/1
  cyemi_143/1 -> cfblk9/1
  cfblk1/1 -> cyemi_143/1
  cyemi_139/1 -> cfblk5/1(emi_1)
  cfblk5/1(emi_2) -> cyemi_136/1
  emi_5/1 -> cfblk5/Action
  emi_5/2 -> emi_3/Action
  emi_6/1 -> emi_5/1
  cyemi_141/1 -> cfblk7/1(emi_78)
  cfblk7/1(emi_79) -> emi_6/1, cyemi_139/1
  emi_82/1 -> cfblk7/Action
  emi_82/2 -> emi_80/Action
  emi_83/1 -> emi_82/1

== system sampleModel7214_pp_1_1_mu/cfblk51 ==
  cfblk1 : Inport
  Action Port : ActionPort  ActionType=else
  cfblk3 : DiscreteStateSpace  SampleTime=-1
  cfblk4 : simulink/Discrete/Transfer Fcn Real Zero  ZeroZ=0.75  ICPrevInput=0.0  DoSatur=off
      settings: SourceProductName=Simulink  SourceProductBaseCode=SL
  cfblk5 : simulink/Discrete/Tapped Delay  vinit=0.0  samptime=-1  NumDelays=1  DelayOrder=Oldest  includeCurrent=off
  cfblk6 : Delay  DelayLengthSource=Input port
      settings: InputPortMap=u0,p1
  cfblk7 : simulink/Continuous/PID Controller  Controller=PID  TimeDomain=Discrete-time  SampleTime=-1  IntegratorMethod=Forward Euler  FilterMethod=Forward Euler  Form=Parallel  UseFilter=on  ControllerParametersSource=internal  P=1  I=1  D=0  N=100  InitialConditionSource=internal  InitialConditionForIntegrator=0  InitialConditionForFilter=0  ExternalReset=none  LimitOutput=off  UpperSaturationLimit=inf  LowerSaturationLimit=-inf  LinearizeAsGain=off  AntiWindupMode=none  Kb=1  TrackingMode=off  Kt=1  PParamMin=[]  PParamMax=[]  IParamMin=[]  IParamMax=[]  DParamMin=[]  DParamMax=[]  NParamMin=[]  NParamMax=[]  KbParamMin=[]  KbParamMax=[]  KtParamMin=[]  KtParamMax=[]  POutMin=[]  POutMax=[]  IOutMin=[]  IOutMax=[]  DOutMin=[]  DOutMax=[]  NOutMin=[]  NOutMax=[]  KbOutMin=[]  KbOutMax=[]  KtOutMin=[]  KtOutMax=[]  IntegratorOutMin=[]  IntegratorOutMax=[]  FilterOutMin=[]  FilterOutMax=[]  SumOutMin=[]  SumOutMax=[]  SumI1OutMin=[]  SumI1OutMax=[]  SumI2OutMin=[]  SumI2OutMax=[]  SumI3OutMin=[]  SumI3OutMax=[]  SumDOutMin=[]  SumDOutMax=[]  SaturationOutMin=[]  SaturationOutMax=[]  IntegratorContinuousStateAttributes=''  IntegratorStateMustResolveToSignalObject=off  IntegratorRTWStateStorageClass=Auto  FilterContinuousStateAttributes=''  FilterStateMustResolveToSignalObject=off  FilterRTWStateStorageClass=Auto  DifferentiatorICPrevScaledInput=0  DifferentiatorOutMin=[]  DifferentiatorOutMax=[]  FilterDiffOutCoefMin=[]  FilterDiffOutCoefMax=[]  SumDenOutMin=[]  SumDenOutMax=[]  SumNumOutMin=[]  SumNumOutMax=[]  ReciprocalOutMin=[]  ReciprocalOutMax=[]  DivideOutMin=[]  DivideOutMax=[]  TunerSelectOption=Transfer Function Based (PID Tuner App)
  cfblk9 : Delay
  cyemi_{145..151} (7 alike) : DataTypeConversion  OutDataTypeStr=double
  cfblk2 : Outport
  cfblk8 : Outport  Port=2
  wires:
  cfblk5/1 -> cfblk2/1, cyemi_151/1
  cfblk7/1 -> cfblk8/1
  cyemi_145/1 -> cfblk3/1
  cfblk9/1 -> cyemi_145/1
  cyemi_146/1 -> cfblk4/1
  cfblk6/1 -> cyemi_146/1
  cyemi_147/1 -> cfblk5/1
  cfblk3/1 -> cyemi_147/1
  cyemi_148/1 -> cfblk6/1
  cfblk1/1 -> cyemi_148/1, cyemi_149/1
  cyemi_149/1 -> cfblk6/2
  cyemi_150/1 -> cfblk7/1
  cfblk4/1 -> cyemi_150/1
  cyemi_151/1 -> cfblk9/1

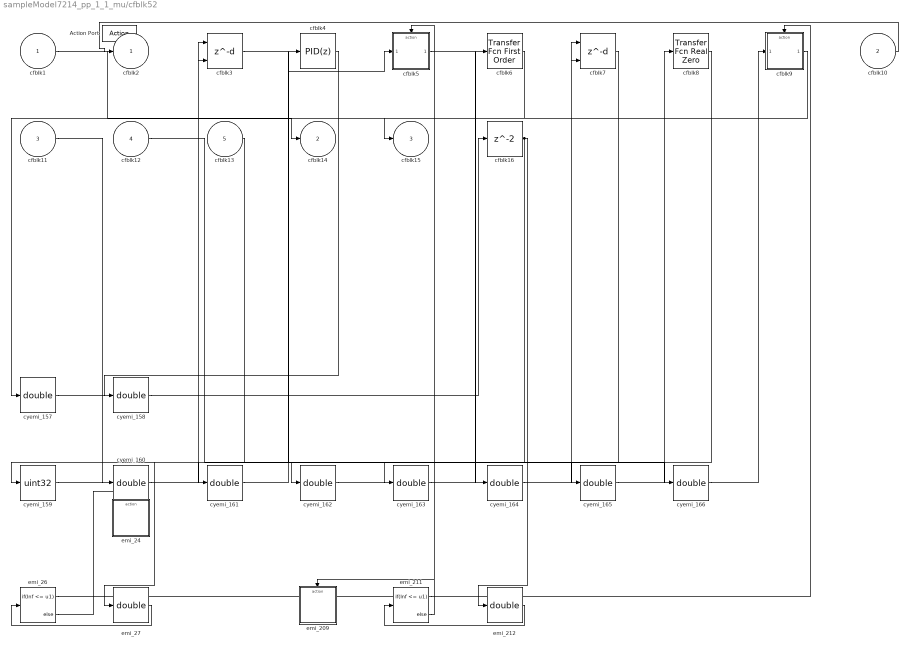
== system sampleModel7214_pp_1_1_mu/cfblk52 ==
  cfblk1 : Inport
  cfblk10 : Inport  Port=2
  cfblk11 : Inport  Port=3
  cfblk12 : Inport  Port=4
  cfblk13 : Inport  Port=5
  Action Port : ActionPort  ActionType=then
  cfblk16 : Delay
  cfblk3 : Delay  DelayLengthSource=Input port
      settings: InputPortMap=u0,p1
  cfblk4 : simulink/Continuous/PID Controller  Controller=PID  TimeDomain=Discrete-time  SampleTime=-1  IntegratorMethod=Forward Euler  FilterMethod=Forward Euler  Form=Parallel  UseFilter=on  ControllerParametersSource=internal  P=1  I=1  D=0  N=100  InitialConditionSource=internal  InitialConditionForIntegrator=0  InitialConditionForFilter=0  ExternalReset=none  LimitOutput=off  UpperSaturationLimit=inf  LowerSaturationLimit=-inf  LinearizeAsGain=off  AntiWindupMode=none  Kb=1  TrackingMode=off  Kt=1  PParamMin=[]  PParamMax=[]  IParamMin=[]  IParamMax=[]  DParamMin=[]  DParamMax=[]  NParamMin=[]  NParamMax=[]  KbParamMin=[]  KbParamMax=[]  KtParamMin=[]  KtParamMax=[]  POutMin=[]  POutMax=[]  IOutMin=[]  IOutMax=[]  DOutMin=[]  DOutMax=[]  NOutMin=[]  NOutMax=[]  KbOutMin=[]  KbOutMax=[]  KtOutMin=[]  KtOutMax=[]  IntegratorOutMin=[]  IntegratorOutMax=[]  FilterOutMin=[]  FilterOutMax=[]  SumOutMin=[]  SumOutMax=[]  SumI1OutMin=[]  SumI1OutMax=[]  SumI2OutMin=[]  SumI2OutMax=[]  SumI3OutMin=[]  SumI3OutMax=[]  SumDOutMin=[]  SumDOutMax=[]  SaturationOutMin=[]  SaturationOutMax=[]  IntegratorContinuousStateAttributes=''  IntegratorStateMustResolveToSignalObject=off  IntegratorRTWStateStorageClass=Auto  FilterContinuousStateAttributes=''  FilterStateMustResolveToSignalObject=off  FilterRTWStateStorageClass=Auto  DifferentiatorICPrevScaledInput=0  DifferentiatorOutMin=[]  DifferentiatorOutMax=[]  FilterDiffOutCoefMin=[]  FilterDiffOutCoefMax=[]  SumDenOutMin=[]  SumDenOutMax=[]  SumNumOutMin=[]  SumNumOutMax=[]  ReciprocalOutMin=[]  ReciprocalOutMax=[]  DivideOutMin=[]  DivideOutMax=[]  TunerSelectOption=Transfer Function Based (PID Tuner App)
  cfblk5 : Subsystem  TreatAsAtomicUnit=on
  cfblk6 : simulink/Discrete/Transfer Fcn First Order  PoleZ=0.95  ICPrevOutput=0.0  DoSatur=off
      settings: SourceProductName=Simulink
  cfblk7 : Delay  DelayLengthSource=Input port
      settings: InputPortMap=u0,p1
  cfblk8 : simulink/Discrete/Transfer Fcn Real Zero  ZeroZ=0.75  ICPrevInput=0.0  DoSatur=off
      settings: SourceProductName=Simulink  SourceProductBaseCode=SL
  cfblk9 : Subsystem  TreatAsAtomicUnit=on
  cyemi_{157..158,160..166} (9 alike) : DataTypeConversion  OutDataTypeStr=double
  cyemi_159 : DataTypeConversion  OutDataTypeStr=uint32
  emi_209 : Subsystem  TreatAsAtomicUnit=on
  emi_211 : If  IfExpression=Inf <= u1
  emi_212 : DataTypeConversion  OutDataTypeStr=double
  emi_24 : Subsystem  TreatAsAtomicUnit=on
  emi_26 : If  IfExpression=Inf <= u1
  emi_27 : DataTypeConversion  OutDataTypeStr=double
  cfblk2 : Outport
  cfblk14 : Outport  Port=2
  cfblk15 : Outport  Port=3
  wires:
  cfblk1/1 -> cfblk14/1
  cfblk10/1 -> cfblk2/1
  cyemi_157/1 -> cfblk16/1
  cfblk6/1 -> cyemi_157/1
  cyemi_158/1 -> cfblk3/1
  cfblk4/1 -> cyemi_158/1
  cyemi_159/1 -> cfblk3/2
  cfblk13/1 -> cyemi_159/1
  cyemi_160/1 -> cfblk4/1
  cfblk11/1 -> cyemi_160/1
  cfblk8/1 -> cyemi_161/1
  cyemi_162/1 -> cfblk6/1
  cfblk7/1 -> cyemi_162/1
  cyemi_163/1 -> cfblk7/1
  cfblk16/1 -> cyemi_163/1, emi_27/1, emi_212/1
  cyemi_164/1 -> cfblk7/2
  cyemi_165/1 -> cfblk8/1
  cfblk12/1 -> cyemi_165/1
  cfblk3/1 -> cyemi_166/1
  cyemi_166/1 -> cfblk9/1(emi_22)
  cfblk9/1(emi_23) -> cfblk15/1
  emi_26/1 -> cfblk9/Action
  emi_26/2 -> emi_24/Action
  emi_27/1 -> emi_26/1
  cyemi_161/1 -> cfblk5/1(emi_207)
  cfblk5/1(emi_208) -> cyemi_164/1
  emi_211/1 -> cfblk5/Action
  emi_211/2 -> emi_209/Action
  emi_212/1 -> emi_211/1

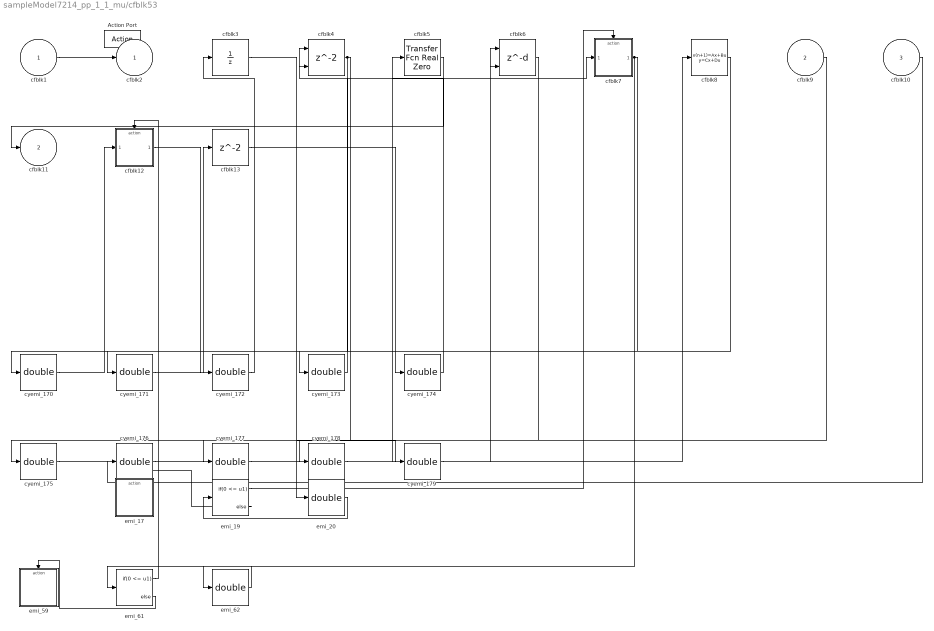
== system sampleModel7214_pp_1_1_mu/cfblk53 ==
  cfblk1 : Inport
  cfblk9 : Inport  Port=2
  cfblk10 : Inport  Port=3
  Action Port : ActionPort  ActionType=else
  cfblk12 : Subsystem  TreatAsAtomicUnit=on
  cfblk13 : Delay
  cfblk3 : UnitDelay  SampleTime=-1
  cfblk4 : Delay  ShowEnablePort=on
      settings: InputPortMap=u0,e6
  cfblk5 : simulink/Discrete/Transfer Fcn Real Zero  ZeroZ=0.75  ICPrevInput=0.0  DoSatur=off
      settings: SourceProductName=Simulink  SourceProductBaseCode=SL
  cfblk6 : Delay  DelayLengthSource=Input port
      settings: InputPortMap=u0,p1
  cfblk7 : Subsystem  TreatAsAtomicUnit=on
  cfblk8 : DiscreteStateSpace  SampleTime=-1
  cyemi_{170..179} (10 alike) : DataTypeConversion  OutDataTypeStr=double
  emi_17 : Subsystem  TreatAsAtomicUnit=on
  emi_19 : If  IfExpression=0 <= u1
  emi_20 : DataTypeConversion  OutDataTypeStr=double
  emi_59 : Subsystem  TreatAsAtomicUnit=on
  emi_61 : If  IfExpression=0 <= u1
  emi_62 : DataTypeConversion  OutDataTypeStr=double
  cfblk2 : Outport
  cfblk11 : Outport  Port=2
  wires:
  cfblk1/1 -> cfblk2/1
  cfblk5/1 -> cfblk11/1
  cyemi_171/1 -> cfblk13/1
  cyemi_172/1 -> cfblk3/1
  cyemi_173/1 -> cfblk4/1
  cfblk8/1 -> cyemi_173/1
  cyemi_174/1 -> cfblk4/2
  cfblk13/1 -> cyemi_174/1
  cyemi_175/1 -> cfblk5/1
  cfblk6/1 -> cyemi_175/1
  cyemi_176/1 -> cfblk6/1
  cfblk10/1 -> cyemi_176/1
  cyemi_177/1 -> cfblk6/2
  cfblk9/1 -> cyemi_177/1
  cfblk4/1 -> cyemi_178/1, emi_20/1
  cyemi_179/1 -> cfblk8/1
  cfblk3/1 -> cyemi_179/1
  cyemi_178/1 -> cfblk7/1(emi_15)
  cfblk7/1(emi_16) -> cyemi_171/1, cyemi_170/1, emi_62/1
  emi_19/1 -> cfblk7/Action
  emi_19/2 -> emi_17/Action
  emi_20/1 -> emi_19/1
  cyemi_170/1 -> cfblk12/1(emi_57)
  cfblk12/1(emi_58) -> cyemi_172/1
  emi_61/1 -> cfblk12/Action
  emi_61/2 -> emi_59/Action
  emi_62/1 -> emi_61/1

== system sampleModel7214_pp_1_1_mu/cfblk60 ==
  emi_171 : Inport
  Action Port : ActionPort  ActionType=then
  cfblk60 : Delay  SampleTime=1
  emi_172 : Outport
  wires:
  emi_171/1 -> cfblk60/1
  cfblk60/1 -> emi_172/1

== system sampleModel7214_pp_1_1_mu/cfblk7 ==
  emi_192 : Inport
  emi_193 : Inport  Port=2
  Action Port : ActionPort  ActionType=then
  cfblk7 : Delay  ShowEnablePort=on  SampleTime=1
      settings: InputPortMap=u0,e6
  emi_194 : Outport
  wires:
  emi_192/1 -> cfblk7/1
  emi_193/1 -> cfblk7/2
  cfblk7/1 -> emi_194/1

== system sampleModel7214_pp_1_1_mu/emi_117 ==
  Action Port : ActionPort  ActionType=else
  emi_118 : Assertion

== system sampleModel7214_pp_1_1_mu/emi_145 ==
  Action Port : ActionPort  ActionType=else
  emi_146 : Assertion

== system sampleModel7214_pp_1_1_mu/emi_173 ==
  Action Port : ActionPort  ActionType=else
  emi_174 : Assertion

== system sampleModel7214_pp_1_1_mu/emi_195 ==
  Action Port : ActionPort  ActionType=else
  emi_196 : Assertion

== system sampleModel7214_pp_1_1_mu/emi_88 ==
  Action Port : ActionPort  ActionType=else
  emi_89 : Assertion

== system sampleModel7214_pp_1_1_mu/emi_95 ==
  Action Port : ActionPort  ActionType=else
  emi_96 : Assertion

== system sampleModel7214_pp_1_1_mu/cfblk46/cfblk7 ==
  emi_43 : Inport
  Action Port : ActionPort  ActionType=then
  cfblk7 : UnitDelay  SampleTime=-1
  emi_44 : Outport
  wires:
  emi_43/1 -> cfblk7/1
  cfblk7/1 -> emi_44/1

== system sampleModel7214_pp_1_1_mu/cfblk46/emi_45 ==
  Action Port : ActionPort  ActionType=else
  emi_46 : Assertion

== system sampleModel7214_pp_1_1_mu/cfblk47/cfblk6 ==
  emi_136 : Inport
  Action Port : ActionPort  ActionType=then
  cfblk6 : simulink/Discrete/Transfer Fcn First Order  PoleZ=0.95  ICPrevOutput=0.0  DoSatur=off
      settings: SourceProductName=Simulink
  emi_137 : Outport
  wires:
  emi_136/1 -> cfblk6/1
  cfblk6/1 -> emi_137/1

== system sampleModel7214_pp_1_1_mu/cfblk47/cfblk8 ==
  emi_129 : Inport
  Action Port : ActionPort  ActionType=then
  cfblk8 : simulink/Discrete/Transfer Fcn Lead or Lag  PoleZ=0.95  ZeroZ=0.75  ICPrevOutput=0.0  ICPrevInput=0.0  DoSatur=off
      settings: SourceProductName=Simulink  SourceProductBaseCode=SL
  emi_130 : Outport
  wires:
  emi_129/1 -> cfblk8/1
  cfblk8/1 -> emi_130/1

== system sampleModel7214_pp_1_1_mu/cfblk47/emi_131 ==
  Action Port : ActionPort  ActionType=else
  emi_132 : Assertion

== system sampleModel7214_pp_1_1_mu/cfblk47/emi_138 ==
  Action Port : ActionPort  ActionType=else
  emi_139 : Assertion

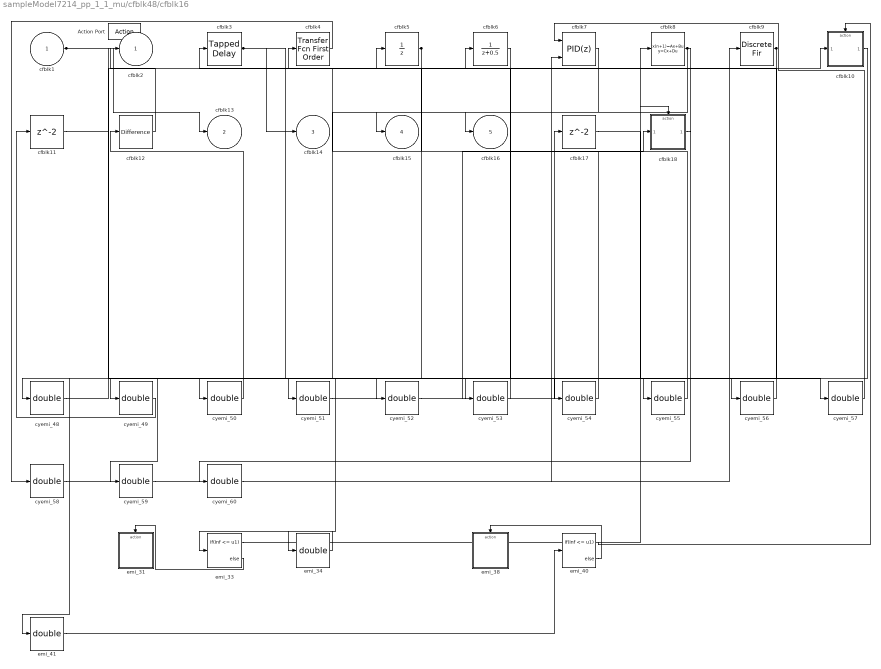
== system sampleModel7214_pp_1_1_mu/cfblk48/cfblk16 ==
  cfblk1 : Inport
  Action Port : ActionPort  ActionType=then
  cfblk10 : Subsystem  TreatAsAtomicUnit=on
  cfblk11 : Delay
  cfblk12 : simulink/Discrete/Difference  ICPrevInput=0.0  OutMin=[]  OutMax=[]  OutDataTypeStr=double  OutputDataTypeScalingMode=double  OutDataType=fixdt(1, 16)  OutScaling=2^-10  DoSatur=off
  cfblk17 : Delay
  cfblk18 : Subsystem  TreatAsAtomicUnit=on
  cfblk3 : simulink/Discrete/Tapped Delay  vinit=0.0  samptime=-1  NumDelays=1  DelayOrder=Oldest  includeCurrent=off
  cfblk4 : simulink/Discrete/Transfer Fcn First Order  PoleZ=0.95  ICPrevOutput=0.0  DoSatur=off
      settings: SourceProductName=Simulink
  cfblk5 : UnitDelay  SampleTime=-1
  cfblk6 : DiscreteTransferFcn
  cfblk7 : simulink/Continuous/PID Controller (2DOF)  Controller=PID  TimeDomain=Discrete-time  SampleTime=-1  IntegratorMethod=Forward Euler  FilterMethod=Forward Euler  Form=Parallel  UseFilter=on  ControllerParametersSource=internal  P=1  I=1  D=0  N=100  b=1  c=1  InitialConditionSource=internal  InitialConditionForIntegrator=0  InitialConditionForFilter=0  ExternalReset=none  LimitOutput=off  UpperSaturationLimit=inf  LowerSaturationLimit=-inf  LinearizeAsGain=off  AntiWindupMode=none  Kb=1  TrackingMode=off  Kt=1  PParamMin=[]  PParamMax=[]  IParamMin=[]  IParamMax=[]  DParamMin=[]  DParamMax=[]  NParamMin=[]  NParamMax=[]  bParamMin=[]  bParamMax=[]  cParamMin=[]  cParamMax=[]  KbParamMin=[]  KbParamMax=[]  KtParamMin=[]  KtParamMax=[]  POutMin=[]  POutMax=[]  IOutMin=[]  IOutMax=[]  DOutMin=[]  DOutMax=[]  NOutMin=[]  NOutMax=[]  bOutMin=[]  bOutMax=[]  cOutMin=[]  cOutMax=[]  KbOutMin=[]  KbOutMax=[]  KtOutMin=[]  KtOutMax=[]  IntegratorOutMin=[]  IntegratorOutMax=[]  FilterOutMin=[]  FilterOutMax=[]  SumOutMin=[]  SumOutMax=[]  Sum1OutMin=[]  Sum1OutMax=[]  Sum2OutMin=[]  Sum2OutMax=[]  Sum3OutMin=[]  Sum3OutMax=[]  SumI1OutMin=[]  SumI1OutMax=[]  SumI2OutMin=[]  SumI2OutMax=[]  SumI3OutMin=[]  SumI3OutMax=[]  SumDOutMin=[]  SumDOutMax=[]  SaturationOutMin=[]  SaturationOutMax=[]  IntegratorContinuousStateAttributes=''  IntegratorStateMustResolveToSignalObject=off  IntegratorRTWStateStorageClass=Auto  FilterContinuousStateAttributes=''  FilterStateMustResolveToSignalObject=off  FilterRTWStateStorageClass=Auto  DifferentiatorICPrevScaledInput=0  DifferentiatorOutMin=[]  DifferentiatorOutMax=[]  FilterDiffOutCoefMin=[]  FilterDiffOutCoefMax=[]  SumDenOutMin=[]  SumDenOutMax=[]  SumNumOutMin=[]  SumNumOutMax=[]  ReciprocalOutMin=[]  ReciprocalOutMax=[]  DivideOutMin=[]  DivideOutMax=[]  TunerSelectOption=Transfer Function Based (PID Tuner App)
  cfblk8 : DiscreteStateSpace  SampleTime=-1
  cfblk9 : DiscreteFir
  cyemi_{48..60} (13 alike) : DataTypeConversion  OutDataTypeStr=double
  emi_31 : Subsystem  TreatAsAtomicUnit=on
  emi_33 : If  IfExpression=Inf <= u1
  emi_34 : DataTypeConversion  OutDataTypeStr=double
  emi_38 : Subsystem  TreatAsAtomicUnit=on
  emi_40 : If  IfExpression=Inf <= u1
  emi_41 : DataTypeConversion  OutDataTypeStr=double
  cfblk2 : Outport
  cfblk13 : Outport  Port=2
  cfblk14 : Outport  Port=3
  cfblk15 : Outport  Port=4
  cfblk16 : Outport  Port=5
  wires:
  cfblk5/1 -> cfblk15/1, emi_34/1
  cfblk8/1 -> cyemi_51/1, cyemi_55/1
  cfblk1/1 -> cfblk13/1, cyemi_53/1
  cfblk3/1 -> cfblk14/1, cyemi_57/1
  cfblk7/1 -> cfblk16/1
  cfblk9/1 -> cyemi_48/1, cyemi_49/1, cyemi_54/1, emi_41/1
  cfblk12/1 -> cfblk2/1
  cyemi_49/1 -> cfblk11/1
  cyemi_50/1 -> cfblk12/1
  cyemi_51/1 -> cfblk17/1
  cfblk11/1 -> cyemi_52/1
  cyemi_53/1 -> cfblk3/1
  cyemi_54/1 -> cfblk4/1
  cyemi_55/1 -> cfblk5/1
  cyemi_56/1 -> cfblk6/1
  cfblk17/1 -> cyemi_56/1
  cyemi_57/1 -> cfblk7/1
  cyemi_58/1 -> cfblk7/2
  cfblk4/1 -> cyemi_58/1
  cyemi_59/1 -> cfblk8/1
  cfblk6/1 -> cyemi_59/1
  cyemi_60/1 -> cfblk9/1
  cyemi_52/1 -> cfblk18/1(emi_29)
  cfblk18/1(emi_30) -> cyemi_60/1
  emi_33/1 -> cfblk18/Action
  emi_33/2 -> emi_31/Action
  emi_34/1 -> emi_33/1
  cyemi_48/1 -> cfblk10/1(emi_36)
  cfblk10/1(emi_37) -> cyemi_50/1
  emi_40/1 -> cfblk10/Action
  emi_40/2 -> emi_38/Action
  emi_41/1 -> emi_40/1

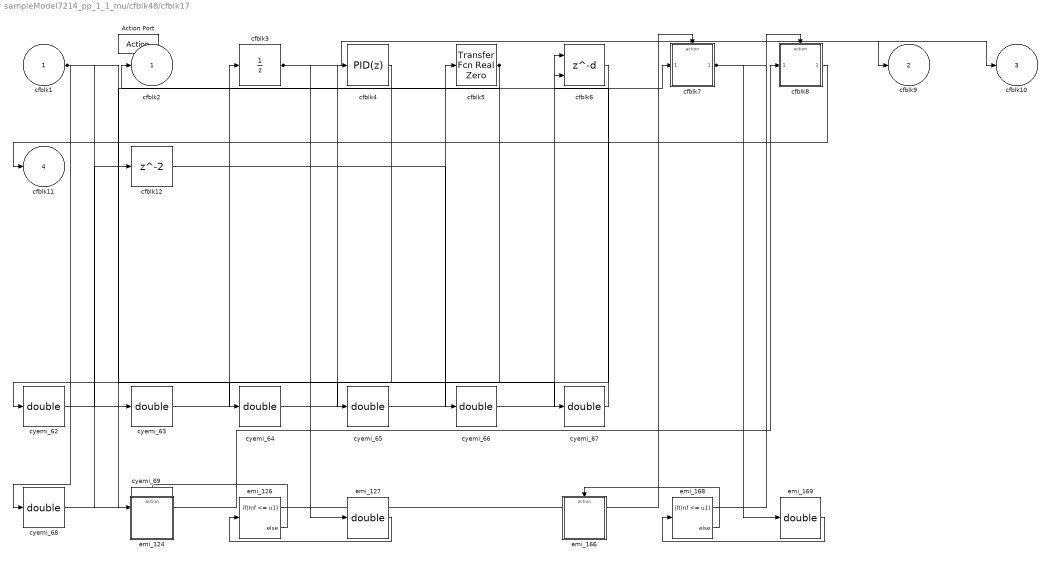
== system sampleModel7214_pp_1_1_mu/cfblk48/cfblk17 ==
  cfblk1 : Inport
  Action Port : ActionPort  ActionType=else
  cfblk12 : Delay
  cfblk3 : UnitDelay  SampleTime=-1
  cfblk4 : simulink/Continuous/PID Controller  Controller=PID  TimeDomain=Discrete-time  SampleTime=-1  IntegratorMethod=Forward Euler  FilterMethod=Forward Euler  Form=Parallel  UseFilter=on  ControllerParametersSource=internal  P=1  I=1  D=0  N=100  InitialConditionSource=internal  InitialConditionForIntegrator=0  InitialConditionForFilter=0  ExternalReset=none  LimitOutput=off  UpperSaturationLimit=inf  LowerSaturationLimit=-inf  LinearizeAsGain=off  AntiWindupMode=none  Kb=1  TrackingMode=off  Kt=1  PParamMin=[]  PParamMax=[]  IParamMin=[]  IParamMax=[]  DParamMin=[]  DParamMax=[]  NParamMin=[]  NParamMax=[]  KbParamMin=[]  KbParamMax=[]  KtParamMin=[]  KtParamMax=[]  POutMin=[]  POutMax=[]  IOutMin=[]  IOutMax=[]  DOutMin=[]  DOutMax=[]  NOutMin=[]  NOutMax=[]  KbOutMin=[]  KbOutMax=[]  KtOutMin=[]  KtOutMax=[]  IntegratorOutMin=[]  IntegratorOutMax=[]  FilterOutMin=[]  FilterOutMax=[]  SumOutMin=[]  SumOutMax=[]  SumI1OutMin=[]  SumI1OutMax=[]  SumI2OutMin=[]  SumI2OutMax=[]  SumI3OutMin=[]  SumI3OutMax=[]  SumDOutMin=[]  SumDOutMax=[]  SaturationOutMin=[]  SaturationOutMax=[]  IntegratorContinuousStateAttributes=''  IntegratorStateMustResolveToSignalObject=off  IntegratorRTWStateStorageClass=Auto  FilterContinuousStateAttributes=''  FilterStateMustResolveToSignalObject=off  FilterRTWStateStorageClass=Auto  DifferentiatorICPrevScaledInput=0  DifferentiatorOutMin=[]  DifferentiatorOutMax=[]  FilterDiffOutCoefMin=[]  FilterDiffOutCoefMax=[]  SumDenOutMin=[]  SumDenOutMax=[]  SumNumOutMin=[]  SumNumOutMax=[]  ReciprocalOutMin=[]  ReciprocalOutMax=[]  DivideOutMin=[]  DivideOutMax=[]  TunerSelectOption=Transfer Function Based (PID Tuner App)
  cfblk5 : simulink/Discrete/Transfer Fcn Real Zero  ZeroZ=0.75  ICPrevInput=0.0  DoSatur=off
      settings: SourceProductName=Simulink  SourceProductBaseCode=SL
  cfblk6 : Delay  DelayLengthSource=Input port
      settings: InputPortMap=u0,p1
  cfblk7 : Subsystem  TreatAsAtomicUnit=on
  cfblk8 : Subsystem  TreatAsAtomicUnit=on
  cyemi_{62..69} (8 alike) : DataTypeConversion  OutDataTypeStr=double
  emi_124 : Subsystem  TreatAsAtomicUnit=on
  emi_126 : If  IfExpression=Inf <= u1
  emi_127 : DataTypeConversion  OutDataTypeStr=double
  emi_166 : Subsystem  TreatAsAtomicUnit=on
  emi_168 : If  IfExpression=Inf <= u1
  emi_169 : DataTypeConversion  OutDataTypeStr=double
  cfblk2 : Outport
  cfblk9 : Outport  Port=2
  cfblk10 : Outport  Port=3
  cfblk11 : Outport  Port=4
  wires:
  cfblk3/1 -> cfblk9/1, emi_127/1
  cfblk1/1 -> cyemi_63/1, cyemi_67/1, cyemi_68/1, cyemi_69/1
  cfblk5/1 -> cfblk2/1, cyemi_62/1
  cyemi_62/1 -> cfblk12/1
  cyemi_63/1 -> cfblk3/1
  cyemi_64/1 -> cfblk4/1
  cfblk6/1 -> cyemi_64/1
  cyemi_65/1 -> cfblk5/1
  cfblk4/1 -> cyemi_65/1
  cyemi_66/1 -> cfblk6/1
  cfblk12/1 -> cyemi_66/1
  cyemi_67/1 -> cfblk6/2
  cyemi_68/1 -> cfblk7/1(emi_122)
  cfblk7/1(emi_123) -> cfblk10/1, emi_169/1
  emi_126/1 -> cfblk7/Action
  emi_126/2 -> emi_124/Action
  emi_127/1 -> emi_126/1
  cyemi_69/1 -> cfblk8/1(emi_164)
  cfblk8/1(emi_165) -> cfblk11/1
  emi_168/1 -> cfblk8/Action
  emi_168/2 -> emi_166/Action
  emi_169/1 -> emi_168/1

== system sampleModel7214_pp_1_1_mu/cfblk48/cfblk4 ==
  emi_108 : Inport
  Action Port : ActionPort  ActionType=then
  cfblk4 : DiscreteFilter
  emi_109 : Outport
  wires:
  emi_108/1 -> cfblk4/1
  cfblk4/1 -> emi_109/1

== system sampleModel7214_pp_1_1_mu/cfblk48/cfblk7 ==
  emi_200 : Inport
  Action Port : ActionPort  ActionType=then
  cfblk7 : DiscreteFir
  emi_201 : Outport
  wires:
  emi_200/1 -> cfblk7/1
  cfblk7/1 -> emi_201/1

== system sampleModel7214_pp_1_1_mu/cfblk48/emi_110 ==
  Action Port : ActionPort  ActionType=else
  emi_111 : Assertion

== system sampleModel7214_pp_1_1_mu/cfblk48/emi_202 ==
  Action Port : ActionPort  ActionType=else
  emi_203 : Assertion

== system sampleModel7214_pp_1_1_mu/cfblk49/cfblk11 ==
  emi_71 : Inport
  Action Port : ActionPort  ActionType=then
  cfblk11 : DiscreteStateSpace  SampleTime=-1
  emi_72 : Outport
  wires:
  emi_71/1 -> cfblk11/1
  cfblk11/1 -> emi_72/1
